simulink model "dynamic_model_step"  (R2021a)
settings: Solver=VariableStepAuto  StartTime=0.0  StopTime=10.0  RelTol=1e-3
undefined symbols (not defined in the file or in its folder): b, g, g_acc, I, Ix, Iy, Iz, k, K_d, k_d, K_i, K_p, L, m
libraries: vrlib x1
settings Model: Creator=filippo  LastModifiedBy=filippo

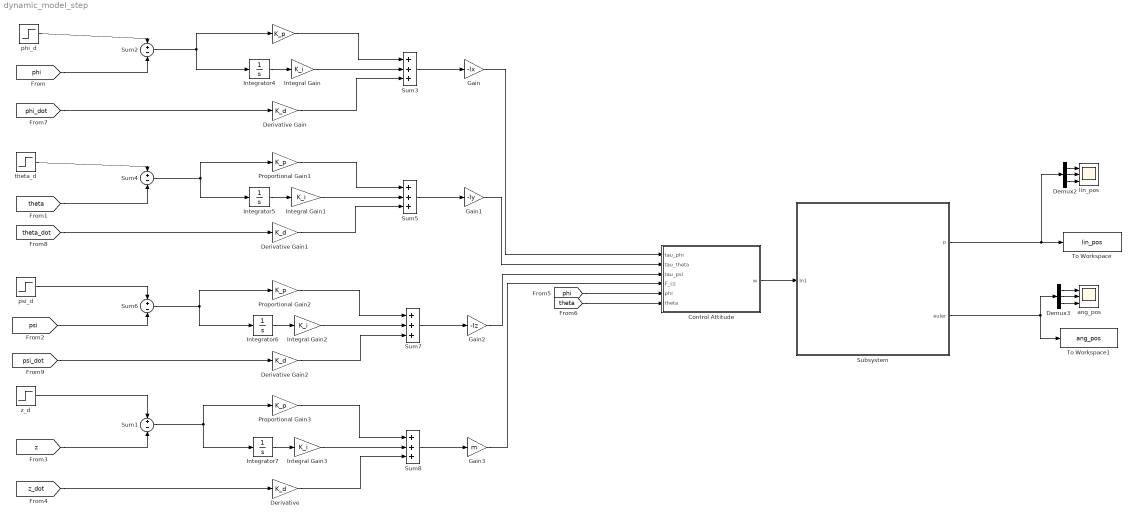
== system dynamic_model_step ==
  " " : Gain  Gain=K_p
  Control Attitude : MATLAB Function  TreatAsAtomicUnit=on
  Demux2 : Demux  Outputs=3
  Demux3 : Demux  Outputs=3
  "Derivative " : Gain  Gain=K_d
  Derivative Gain : Gain  Gain=K_d
  Derivative Gain1 : Gain  Gain=K_d
  Derivative Gain2 : Gain  Gain=K_d
  Gain : Gain  Gain=-Ix
  Gain1 : Gain  Gain=-Iy
  Gain2 : Gain  Gain=-Iz
  Gain3 : Gain  Gain=m
  Integral Gain{,1..3} (4 alike) : Gain  Gain=K_i
  Integrator{4..7} (4 alike) : Integrator
  Proportional Gain1 : Gain  Gain=K_p
  Proportional Gain2 : Gain  Gain=K_p
  Proportional Gain3 : Gain  Gain=K_p
  Subsystem : Subsystem
  Sum{1..2,4,6} (4 alike) : Sum  Inputs=+|-
  Sum{3,5,7..8} (4 alike) : Sum  Inputs=+++
  To Workspace : ToWorkspace  VariableName=lin_pos  SaveFormat=Timeseries  SampleTime=-1
  To Workspace1 : ToWorkspace  VariableName=ang_pos  SaveFormat=Timeseries  SampleTime=-1
  ang_pos : Scope  NumInputPorts=3
  lin_pos : Scope  NumInputPorts=3
  phi_d : Step  After=10  SampleTime=0
  psi_d : Step  After=0  SampleTime=0
  theta_d : Step  After=0  SampleTime=0
  z_d : Step  After=0  SampleTime=0
  wires:
  " "/1 -> Sum3/1
  [theta] -> Control Attitude/6(theta)
  Control Attitude/1(w) -> Subsystem/1(In1)
  Demux3/1 -> ang_pos/1
  Demux3/2 -> ang_pos/2
  theta_d/1 -> Sum4/1
  Sum7/1 -> Gain2/1
  Demux2/3 -> lin_pos/3
  Integrator5/1 -> Integral Gain1/1
  Sum3/1 -> Gain/1
  Gain/1 -> Control Attitude/1(tau_phi)
  Integral Gain3/1 -> Sum8/2
  Subsystem/2(euler) -> To Workspace1/1, Demux3/1
  [phi] -> Sum2/2
  Integrator7/1 -> Integral Gain3/1
  Sum8/1 -> Gain3/1
  Demux2/2 -> lin_pos/2
  Proportional Gain2/1 -> Sum7/1
  [z_dot] -> "Derivative "/1
  psi_d/1 -> Sum6/1
  Proportional Gain1/1 -> Sum5/1
  [psi_dot] -> Derivative Gain2/1
  [phi_dot] -> Derivative Gain/1
  Derivative Gain2/1 -> Sum7/3
  [phi] -> Control Attitude/5(phi)
  Sum5/1 -> Gain1/1
  Subsystem/1(p) -> Demux2/1, To Workspace/1
  Demux2/1 -> lin_pos/1
  z_d/1 -> Sum1/1
  Sum1/1 -> Integrator7/1, Proportional Gain3/1
  Demux3/3 -> ang_pos/3
  Derivative Gain1/1 -> Sum5/3
  Gain1/1 -> Control Attitude/2(tau_theta)
  "Derivative "/1 -> Sum8/3
  [psi] -> Sum6/2
  Integrator4/1 -> Integral Gain/1
  Integral Gain2/1 -> Sum7/2
  Gain3/1 -> Control Attitude/4(F_cz)
  Sum2/1 -> Integrator4/1, " "/1
  Sum6/1 -> Integrator6/1, Proportional Gain2/1
  Integrator6/1 -> Integral Gain2/1
  Integral Gain1/1 -> Sum5/2
  [z] -> Sum1/2
  [theta_dot] -> Derivative Gain1/1
  Integral Gain/1 -> Sum3/2
  phi_d/1 -> Sum2/1
  Proportional Gain3/1 -> Sum8/1
  Derivative Gain/1 -> Sum3/3
  Sum4/1 -> Integrator5/1, Proportional Gain1/1
  Gain2/1 -> Control Attitude/3(tau_psi)
  [theta] -> Sum4/2

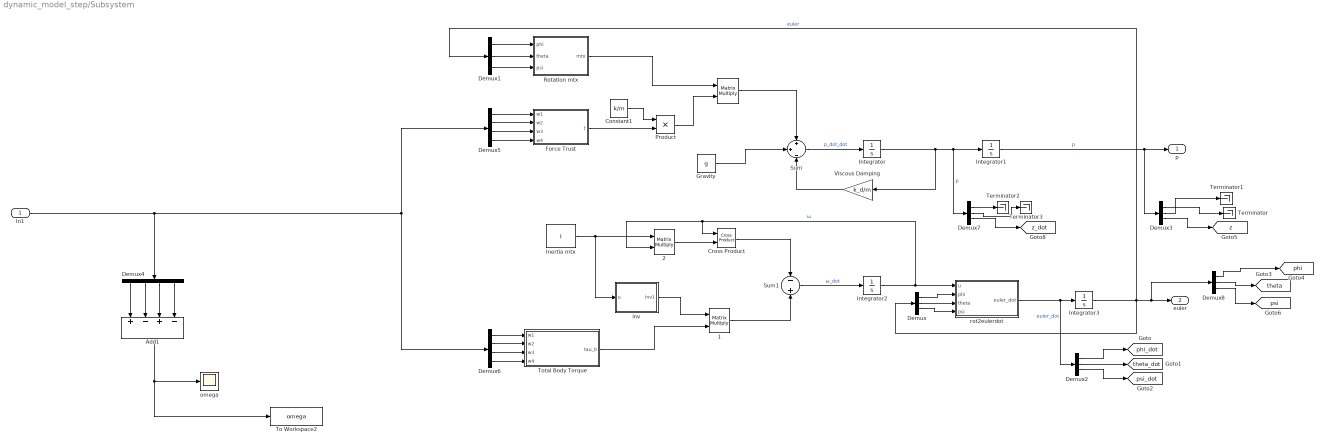
== system dynamic_model_step/Subsystem ==
  In1 : Inport
  " " : Product  Multiplication=Matrix(*)
  " 1" : Product  Multiplication=Matrix(*)
  " 2" : Product  Multiplication=Matrix(*)
  Add1 : Sum  Inputs=+-+-
  Constant1 : Constant  Value=k/m
  Cross Product : vrlib/Utilities/Cross Product
  Demux{,1..3,7..8} (6 alike) : Demux  Outputs=3
  Demux4 : Demux
  Demux5 : Demux
  Demux6 : Demux
  Force Trust : MATLAB Function  TreatAsAtomicUnit=on
  Gravity : Constant  Value=g  VectorParams1D=off
  Inertia mtx : Constant  Value=I  VectorParams1D=off
  Integrator{,1..3} (4 alike) : Integrator
  Product : Product
  Rotation mtx : MATLAB Function  TreatAsAtomicUnit=on
  Sum : Sum  Inputs=+|+|-
  Sum1 : Sum  Inputs=-|+
  Terminator{,1..3} (4 alike) : Terminator
  To Workspace2 : ToWorkspace  VariableName=omega  SaveFormat=Timeseries  SampleTime=-1
  Total Body Torque : MATLAB Function  TreatAsAtomicUnit=on
  Viscous Damping : Gain  Gain=k_d/m
  inv : MATLAB Function  TreatAsAtomicUnit=on
  omega : Scope
  rot2eulerdot : MATLAB Function  TreatAsAtomicUnit=on
  p : Outport
  euler : Outport  Port=2
  tag scope: phi=global, phi_dot=global, psi=global, psi_dot=global, theta=global, theta_dot=global, z=global, z_dot=global
  wires:
  " "/1 -> Sum/1
  " 1"/1 -> Sum1/2
  Constant1/1 -> Product/1
  Sum/1 -> Integrator/1  "p_dot_dot"
  " 2"/1 -> Cross Product/2
  Rotation mtx/1(mtx) -> " "/1
  Demux5/4 -> Force Trust/4(w4)
  Demux4/1 -> Add1/1
  Demux1/3 -> Rotation mtx/3(psi)
  Force Trust/1(f) -> Product/2
  Demux4/3 -> Add1/3
  Demux5/2 -> Force Trust/2(w2)
  Gravity/1 -> Sum/2
  Demux1/1 -> Rotation mtx/1(phi)
  inv/1(inv1) -> " 1"/1
  Demux1/2 -> Rotation mtx/2(theta)
  Demux6/4 -> Total Body Torque/4(w4)
  Demux/2 -> rot2eulerdot/3(theta)
  Sum1/1 -> Integrator2/1  "ω_dot"
  Add1/1 -> To Workspace2/1, omega/1
  Cross Product/1 -> Sum1/1
  Demux4/2 -> Add1/2
  rot2eulerdot/1(euler_dot) -> Demux2/1, Integrator3/1  "euler_dot"
  Product/1 -> " "/2
  Inertia mtx/1 -> " 2"/1, inv/1(u)
  Integrator3/1 -> Demux8/1, euler/1, Demux/1, Demux1/1  "euler"
  Demux/1 -> rot2eulerdot/2(phi)
  Demux5/3 -> Force Trust/3(w3)
  Demux6/1 -> Total Body Torque/1(w1)
  Viscous Damping/1 -> Sum/3
  In1/1 -> Demux6/1, Demux5/1, Demux4/1
  Demux4/4 -> Add1/4
  Integrator2/1 -> rot2eulerdot/1(u), Cross Product/1, " 2"/2  "ω"
  Demux6/3 -> Total Body Torque/3(w3)
  Total Body Torque/1(tau_b) -> " 1"/2
  Demux/3 -> rot2eulerdot/4(psi)
  Demux5/1 -> Force Trust/1(w1)
  Demux6/2 -> Total Body Torque/2(w2)
  Demux2/1 -> [phi_dot]
  Demux2/3 -> [psi_dot]
  Demux2/2 -> [theta_dot]
  Demux3/3 -> [z]
  Integrator1/1 -> Demux3/1, p/1  "p"
  Integrator/1 -> Viscous Damping/1, Demux7/1, Integrator1/1  "p"
  Demux7/3 -> [z_dot]
  Demux3/1 -> Terminator/1
  Demux3/2 -> Terminator1/1
  Demux7/1 -> Terminator2/1
  Demux7/2 -> Terminator3/1
  Demux8/1 -> [phi]
  Demux8/2 -> [theta]
  Demux8/3 -> [psi]

== matlab function dynamic_model_step/Subsystem/Force Trust ==
  data: w1 input; f output [..2]; w2 input; w3 input; w4 input
function f= F_b(w1,w2,w3,w4)
mtx = [0; 0; w1+w2+w3+w4];
f = mtx;
end

== matlab function dynamic_model_step/Subsystem/Rotation mtx ==
  data: phi input; mtx output; theta input; psi input
function mtx = ROTATION(phi, theta, psi)
Rx = [1 0 0; 0 cos(phi) -sin(phi); 0 sin(phi) cos(phi)];
Ry = [cos(theta) 0 sin(theta); 0 1 0; -sin(theta) 0 cos(theta)];
Rz = [cos(psi) -sin(psi) 0; sin(psi) cos(psi) 0; 0 0 1];

% Rot matrix Body-fixed frame wrt Inertial frame
R = Rz * Ry * Rx;
mtx = R;
end

== matlab function dynamic_model_step/Subsystem/Total Body Torque ==
  data: w1 input; tau_b output; w2 input; w3 input; w4 input; L parameter; k parameter; b parameter
function tau_b= TotalBodyTorque(w1, w2, w3, w4, L, k, b)
tau_b = [L*k*(w1-w3); L*k*(w2-w4); b*(w1-w2+w3-w4)];
end

== matlab function dynamic_model_step/Subsystem/inv ==
  data: u input; inv1 output
function inv1 = inv1(u)
% inv = pinv(u);
inv1 = inv(u);
end

== matlab function dynamic_model_step/Subsystem/rot2eulerdot ==
  data: u input; phi input; euler_dot output; theta input; psi input
function euler_dot = rot2euler(u, phi, theta, psi)
R = [1 0 -sin(theta); 0 cos(phi) cos(theta)*sin(phi); 0 -sin(phi) cos(theta)*cos(phi)];
% invR = pinv(R);
invR = inv(R);
euler_dot = invR*u;
end

== matlab function dynamic_model_step/Control Attitude ==
  data: tau_phi input; w output; tau_theta input; tau_psi input; F_cz input; phi input; theta input; L parameter; k parameter; b parameter; m parameter; g_acc parameter
function w = AttitudeControl(tau_phi, tau_theta, tau_psi,F_cz, phi, theta, L, k, b, m, g_acc)
A = [L*k 0 -L*k 0;
    0 L*k 0 -L*k;
    b -b b -b;
    1 1 1 1];
invA = inv(A);
U = [tau_phi;
     tau_theta;
     tau_psi;
     m*g_acc/(k*cos(theta)*cos(phi)) + F_cz];
w = invA*U;
end
